simulink model "Mechanical_System_Simulink"  (R2024a)
settings: Solver=VariableStepAuto  StartTime=0.0  StopTime=10.0  RelTol=1e-3
undefined symbols (not defined in the file): b, bt, F, J, k, kt, m, r
settings Model: Creator=buttrakd  LastModifiedBy=buttrakd

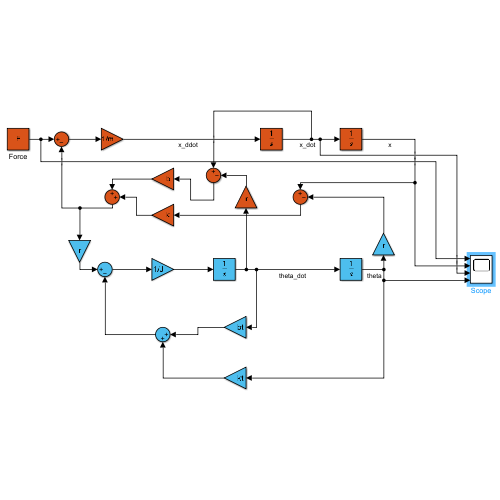
[thumbnail: Simulink's stored preview of the top-level diagram]
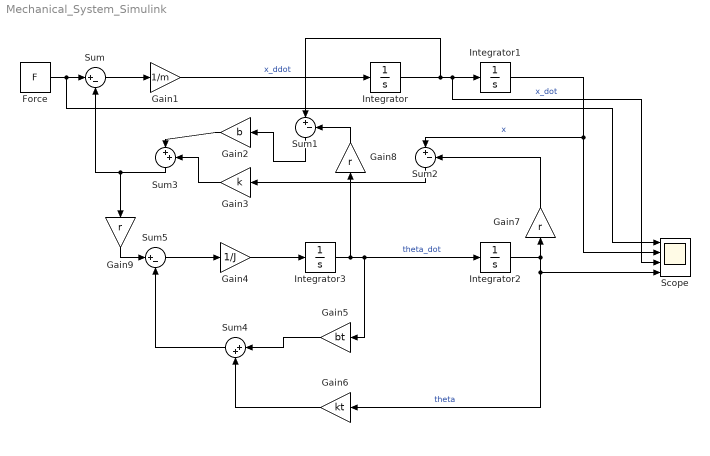
== system Mechanical_System_Simulink ==
  Force : Constant  Value=F
  Gain1 : Gain  Gain=1/m
  Gain2 : Gain  Gain=b
  Gain3 : Gain  Gain=k
  Gain4 : Gain  Gain=1/J
  Gain5 : Gain  Gain=bt
  Gain6 : Gain  Gain=kt
  Gain7 : Gain  Gain=r
  Gain8 : Gain  Gain=r
  Gain9 : Gain  Gain=r
  Integrator{,1..3} (4 alike) : Integrator
  Scope : Scope  NumInputPorts=4
  Sum{,1..2,5} (4 alike) : Sum  Inputs=|+-
  Sum3 : Sum  Inputs=|++
  Sum4 : Sum  Inputs=|++
  wires:
  Integrator/1 -> Scope/3, Integrator1/1, Sum1/1  "x_dot"
  Integrator3/1 -> Gain8/1, Gain5/1, Integrator2/1  "theta_dot"
  Force/1 -> Scope/1, Sum/1
  Sum/1 -> Gain1/1
  Gain1/1 -> Integrator/1  "x_ddot"
  Sum1/1 -> Gain2/1
  Sum2/1 -> Gain3/1
  Gain2/1 -> Sum3/1
  Gain3/1 -> Sum3/2
  Gain4/1 -> Integrator3/1
  Gain5/1 -> Sum4/1
  Gain6/1 -> Sum4/2
  Sum4/1 -> Sum5/2
  Sum3/1 -> Sum/2, Gain9/1
  Integrator2/1 -> Gain6/1, Scope/4, Gain7/1  "theta"
  Gain7/1 -> Sum2/2
  Gain8/1 -> Sum1/2
  Sum5/1 -> Gain4/1
  Gain9/1 -> Sum5/1
  Integrator1/1 -> Scope/2, Sum2/1  "x"
